simulink subsystem "Motor_BAv01"  (R2022b)
settings: Solver=VariableStepAuto  StartTime=0.0  StopTime=10.0  RelTol=1e-3
settings Model: Creator=giaco  LastModifiedBy=giaco

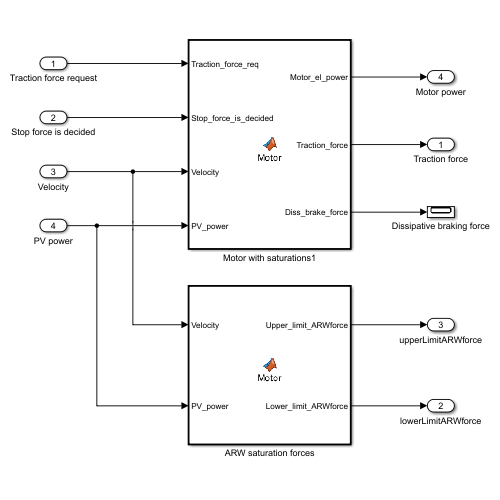
[thumbnail: Simulink's stored preview of the top-level diagram]
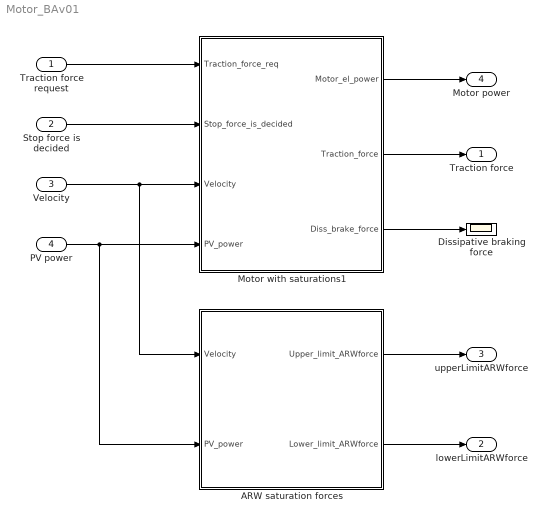
== system Motor_BAv01 ==
  Traction force request : Inport
  Stop force is decided : Inport  Port=2
  Velocity : Inport  Port=3
  PV power : Inport  Port=4
  ARW saturation forces : MATLAB Function  TreatAsAtomicUnit=on
  Dissipative braking force : Scope
  Motor with saturations1 : MATLAB Function  TreatAsAtomicUnit=on
  Traction force : Outport
  lowerLimitARWforce : Outport  Port=2
  upperLimitARWforce : Outport  Port=3
  Motor power : Outport  Port=4
  wires:
  ARW saturation forces/2(Lower_limit_ARWforce) -> lowerLimitARWforce/1
  Motor with saturations1/2(Traction_force) -> Traction force/1
  Motor with saturations1/3(Diss_brake_force) -> Dissipative braking force/1
  Motor with saturations1/1(Motor_el_power) -> Motor power/1
  ARW saturation forces/1(Upper_limit_ARWforce) -> upperLimitARWforce/1
  Stop force is decided/1 -> Motor with saturations1/2(Stop_force_is_decided)
  Traction force request/1 -> Motor with saturations1/1(Traction_force_req)
  Velocity/1 -> ARW saturation forces/1(Velocity), Motor with saturations1/3(Velocity)
  PV power/1 -> ARW saturation forces/2(PV_power), Motor with saturations1/4(PV_power)

== matlab function Motor_BAv01/ARW saturation forces ==
  data: Velocity input; PV_power input; param parameter; Upper_limit_ARWforce output; Lower_limit_ARWforce output
function [Upper_limit_ARWforce, Lower_limit_ARWforce] = Motor(Velocity, PV_power, param)

%% Limits
minElPowerMotBat = param.battery.lowerBoundPower .* param.battery.totNum + PV_power;
minMechPowerMotBat = elPower2mechPower_Willans(minElPowerMotBat, param);

maxElPowerMotBat = param.battery.upperBoundPower .* param.battery.totNum + PV_power;
maxMechPowerMotBat = elPower2mechPower_Willans(maxElPowerMotBat, param);

%% Lower limits
Lower_limit_ARWforce = max(param.motor.minTorque * param.motor.transmissionRatio/param.suspension.rWheel, param.motor.minPower / max(Velocity, 1e-8));
Lower_limit_ARWforce = min(Lower_limit_ARWforce, minMechPowerMotBat / max(Velocity, 1e-8));

%% Upper limits
Upper_limit_ARWforce = min(param.motor.maxTorque * param.motor.transmissionRatio/param.suspension.rWheel, param.motor.maxPower / max(Velocity, 1e-8));
Upper_limit_ARWforce = min(Upper_limit_ARWforce, maxMechPowerMotBat / max(Velocity, 1e-8));

end % fct

== matlab function Motor_BAv01/Motor with saturations1 ==
  data: Traction_force_req input; Stop_force_is_decided input; Velocity input; PV_power input; param parameter; Motor_el_power output; Traction_force output; Diss_brake_force output
function [Motor_el_power, Traction_force, Diss_brake_force] = Motor(Traction_force_req, Stop_force_is_decided, Velocity, PV_power, param)

Diss_brake_force = 0;

%%  Conversion battery limits
minElPowerMotBat = param.battery.lowerBoundPower .* param.battery.totNum + PV_power;
minMechPowerMotBat = elPower2mechPower_Willans(minElPowerMotBat, param);

maxElPowerMotBat = param.battery.upperBoundPower .* param.battery.totNum + PV_power;
maxMechPowerMotBat = elPower2mechPower_Willans(maxElPowerMotBat, param);

%% Standing condition
if Stop_force_is_decided
    Traction_force = 0;
    Motor_el_power = 0;

else
%% Conversions
    tractionTorqueReq = Traction_force_req * param.suspension.rWheel/param.motor.transmissionRatio;
    omegaMot = Velocity * param.motor.transmissionRatio/param.suspension.rWheel;

%% Limits
    tractionTorque = min(tractionTorqueReq, param.motor.maxPower / max(omegaMot, 1e-8)); %upper limit power motor
    tractionTorque = max(tractionTorque, param.motor.minPower / max(omegaMot, 1e-8)); %lower limit power motor
    tractionTorque = min(tractionTorque, maxMechPowerMotBat / max(omegaMot, 1e-8)); %upper limit power battery
    tractionTorque = max(tractionTorque, minMechPowerMotBat / max(omegaMot, 1e-8)); %lower limit power battery
    tractionTorque = min(tractionTorque, param.motor.maxTorque);
    tractionTorque = max(tractionTorque, param.motor.minTorque);
    
%% Electric motor power
    mechPower = omegaMot * tractionTorque;
    Motor_el_power = mechPower2elPower_Willans(mechPower, param);

%% Traction force
    Traction_force = tractionTorque * param.motor.transmissionRatio / param.suspension.rWheel;

    %additional dissipative braking force
    deltaBrake = Traction_force_req - Traction_force;
    if deltaBrake < 0
        Diss_brake_force = deltaBrake;
        Traction_force = Traction_force + Diss_brake_force;
    end % if
end % if
end % fct
